simulink model "VCond_TestBed_org"  (Simulink 10.0)
settings: Solver=FixedStepDiscrete  StartTime=0.0  StopTime=1  FixedStep=1  RelTol=1e-3  EnableMultiTasking=on
undefined symbols (not defined in the file): MWS
libraries: Lib_Solve_VectorCondition_TMATS x1
settings Model: Creator=jwchapm2  LastModifiedBy=bhisma
settings DataIOCC: LimitDataPoints=on
settings OptimizationCC: ExpressionDepthLimit=2147483647
settings DebuggingCC: SolverPrmCheckMsg=warning  StateNameClashWarn=warning
settings GRTTargetCC: GeneratePreprocessorConditionals=Disable all  CombineOutputUpdateFcns=on  GRTInterface=off
settings ConfigComp: CovExternalEMLEnable=off

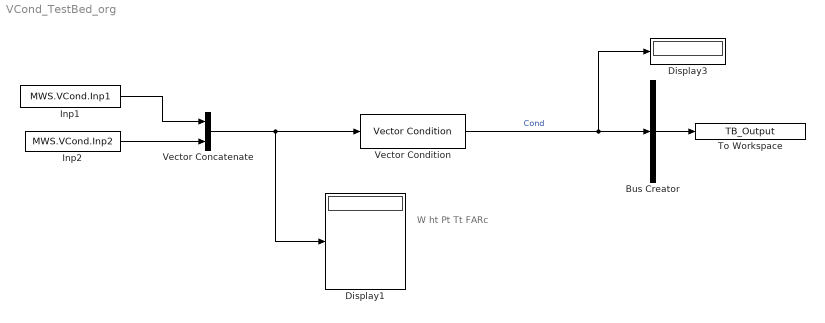
== system VCond_TestBed_org ==
  note: W
      | ht
      | Pt
      | Tt
      | FARc
  Bus Creator : BusCreator  Inputs=1
  Display1 : Display
  Display3 : Display
  Inp1 : Constant  Value=MWS.VCond.Inp1
  Inp2 : Constant  Value=MWS.VCond.Inp2
  To Workspace : ToWorkspace  VariableName=TB_Output  SampleTime=-1
  Vector Concatenate : Concatenate
  Vector Condition : Lib_Solve_VectorCondition_TMATS/Vector Condition  Cond_Limits_M=MWS.VCond.CondLim
  wires:
  Inp1/1 -> Vector Concatenate/1
  Vector Concatenate/1 -> Vector Condition/1, Display1/1
  Vector Condition/1 -> Display3/1, Bus Creator/1  "Cond"
  Bus Creator/1 -> To Workspace/1
  Inp2/1 -> Vector Concatenate/2
